simulink model "Quad_Plant_dynamics"  (R2023b)
settings: Solver=FixedStepAuto  StartTime=0.0  StopTime=10.0  RelTol=1e-3
undefined symbols (not defined in the file): altToPrsBias, altToPrsGain, b, battCapacity, c, contact, dragCoeffMov, fractalcoef, g, mass, ms2_to_mg, ms_to_cms, Payload, rotorDir, rotorPositions, rotorThrustMax, rotorTimeConst, rotorTorqueMax, SampleTime, windVel
libraries: simulink x3, uavmavlinklib x3, sharedtransform x2, robotcorelib x2, sensorinslib x1, shared6dof x1, mspsensorlib x1, uavutilslib x1
(part 1 of 2)
settings Model: Creator=The MathWorks, Inc.  LastModifiedBy=LonelyRetard420
settings SolverCC: AlgebraicLoopSolver=TrustRegion
settings OptimizationCC: ReuseModelBlockBuffer=off
settings DebuggingCC: ParameterPrecisionLossMsg=none  UnconnectedInputMsg=warning  UnconnectedOutputMsg=warning  UnconnectedLineMsg=warning
settings ModelReferenceCC: EnableRefExpFcnMdlSchedulingChecks=on  ModelReferenceNumInstancesAllowed=Single
settings RTWCC: DLArmComputeVersion=19.05

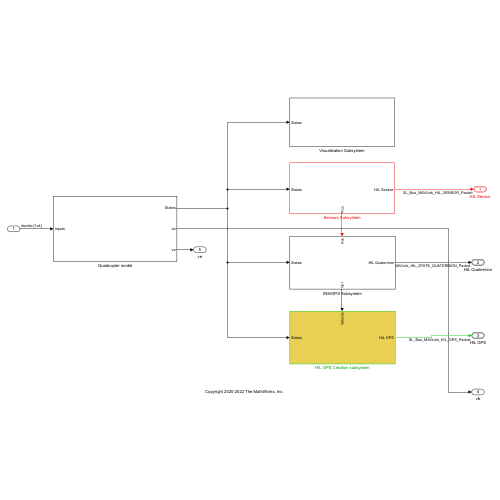
[thumbnail: Simulink's stored preview of the top-level diagram]
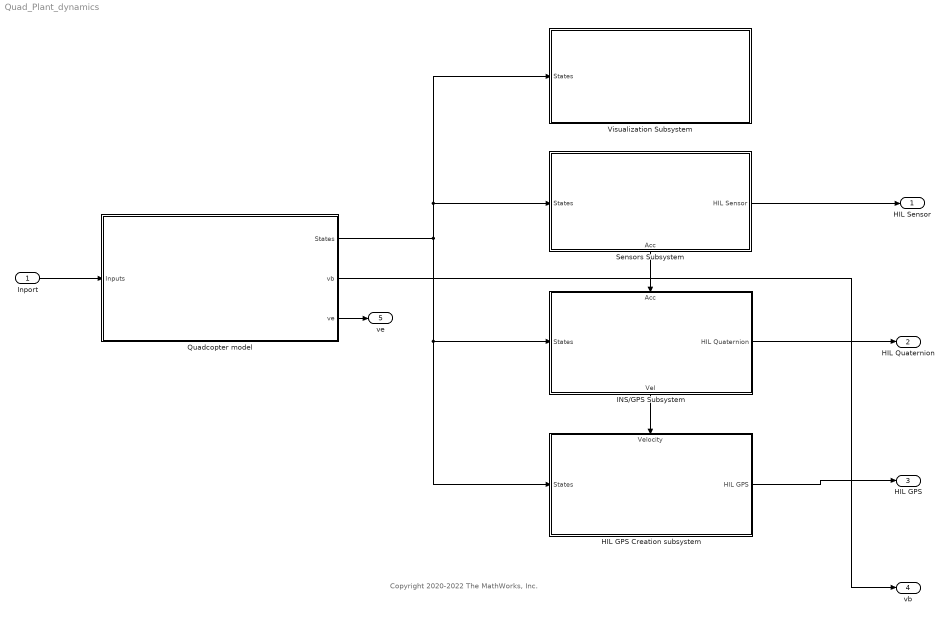
== system Quad_Plant_dynamics ==
  note: Copyright 2020-2022 The MathWorks, Inc.
  Inport : Inport  OutDataTypeStr=double  PortDimensions=[1 4]
  HIL GPS Creation subsystem : Subsystem
      settings: PortSchema="{\"entries\":[{\"content\":{\"sides\":[{\"content\":{\"connectorIds\":[\"In1\"]},\"type\":\"ConnectorPlacement.EquallySpacedRectSide\",\"uuid\":\"f4444677-f205-4bd8-9e95-5e6060697dc4\"},{\"content\":{\"connectorIds\":[\"Out1\"],\"side\":\"RIGHT\"},\"type\":\"ConnectorPlacement.EquallySpacedRectSide\",\"uuid\":\"c948a3e0-826b-4d7b-9e4f-6e3881854d5a\"},{\"content\":{\"connectorIds\":[\"In2\"],\"side\":\"TOP\"},\"type\":\"ConnectorPlacement.EquallySpacedRectSide\",\"uuid\":\"82cf0daf-0b59-4b3c-ab0e-258a514f37ad\"},{\"content\":{\"connectorIds\":[],\"side\":\"HIDDEN\"},\"type\":\"ConnectorPlacement.EquallySpacedRectSide\",\"uuid\":\"a794f320-9150-4c05-acf0-96079b0d3066\"}]},\"type\":\"ConnectorPlacement.EquallySpacedConnector\",\"uuid\":\"8d0915ff-9064-46da-be4f-31886e994f25\"}],\"packageUris\":[\"http://schema.mathworks.com/mf0/Connector/R2020b\"],\"version\":\"1.0\"}"
  INS/GPS Subsystem : Subsystem
      settings: PortSchema="{\"entries\":[{\"content\":{\"sides\":[{\"content\":{\"connectorIds\":[\"In1\"]},\"type\":\"ConnectorPlacement.EquallySpacedRectSide\",\"uuid\":\"bd7d303d-974a-4dd9-8d27-04cf87176bd7\"},{\"content\":{\"connectorIds\":[\"Out1\"],\"side\":\"RIGHT\"},\"type\":\"ConnectorPlacement.EquallySpacedRectSide\",\"uuid\":\"9b60b4cf-af27-4ca7-86b7-e75d27668f15\"},{\"content\":{\"connectorIds\":[\"In2\"],\"side\":\"TOP\"},\"type\":\"ConnectorPlacement.EquallySpacedRectSide\",\"uuid\":\"cd4d20a6-3033-4c65-942d-f02a7fa933e8\"},{\"content\":{\"connectorIds\":[\"Out2\"],\"side\":\"BOTTOM\"},\"type\":\"ConnectorPlacement.EquallySpacedRectSide\",\"uuid\":\"d837ff15-3ee7-4ba9-aab0-0378a7633b3a\"},{\"content\":{\"connectorIds\":[],\"side\":\"HIDDEN\"},\"type\":\"ConnectorPlacement.EquallySpacedRectSide\",\"uuid\":\"eefe2c49-f98f-4c11-8e75-b071b558b610\"}]},\"type\":\"ConnectorPlacement.EquallySpacedConnector\",\"uuid\":\"bd9fca06-cb18-49af-bec9-4d4823ab7b04\"}],\"packageUris\":[\"http://schema.mathworks.com/mf0/Connector/R2020b\"],\"version\":\"1.0\"}"
  Quadcopter model : Subsystem
  Sensors Subsystem : Subsystem
      settings: PortSchema="{\"entries\":[{\"content\":{\"sides\":[{\"content\":{\"connectorIds\":[\"In1\"]},\"type\":\"ConnectorPlacement.EquallySpacedRectSide\",\"uuid\":\"0f5c2282-ad4e-4c27-a92f-532c88dd9b34\"},{\"content\":{\"connectorIds\":[\"Out1\"],\"side\":\"RIGHT\"},\"type\":\"ConnectorPlacement.EquallySpacedRectSide\",\"uuid\":\"b1a389a9-bd19-4f0a-ab56-19663216dbdf\"},{\"content\":{\"connectorIds\":[],\"side\":\"TOP\"},\"type\":\"ConnectorPlacement.EquallySpacedRectSide\",\"uuid\":\"61bb26dd-3b4e-45d7-8996-b1e12f9a0a9d\"},{\"content\":{\"connectorIds\":[\"Out2\"],\"side\":\"BOTTOM\"},\"type\":\"ConnectorPlacement.EquallySpacedRectSide\",\"uuid\":\"ba157af1-2ca4-4452-bdd7-6e3dad9cb5e7\"},{\"content\":{\"connectorIds\":[],\"side\":\"HIDDEN\"},\"type\":\"ConnectorPlacement.EquallySpacedRectSide\",\"uuid\":\"fff182b3-fe96-4082-825e-95746cd3e6b2\"}]},\"type\":\"ConnectorPlacement.EquallySpacedConnector\",\"uuid\":\"8a88afc7-c2a2-4beb-8758-d3390628bed4\"}],\"packageUris\":[\"http://schema.mathworks.com/mf0/Connector/R2020b\"],\"version\":\"1.0\"}"
  Visualization Subsystem : Subsystem
  HIL Sensor : Outport  OutDataTypeStr=Bus: SL_Bus_MAVLink_HIL_SENSOR_Packet  BusOutputAsStruct=on
  HIL Quaternion : Outport  Port=2  OutDataTypeStr=Bus: SL_Bus_MAVLink_HIL_STATE_QUATERNION_Packet  BusOutputAsStruct=on
  HIL GPS : Outport  Port=3  OutDataTypeStr=Bus: SL_Bus_MAVLink_HIL_GPS_Packet  BusOutputAsStruct=on
  vb : Outport  Port=4
  ve : Outport  Port=5
  wires:
  Sensors Subsystem/1(HIL Sensor) -> HIL Sensor/1
  HIL GPS Creation subsystem/1(HIL GPS) -> HIL GPS/1
  INS/GPS Subsystem/2(Vel) -> HIL GPS Creation subsystem/2(Velocity)
  Quadcopter model/1(States) -> HIL GPS Creation subsystem/1(States), INS/GPS Subsystem/1(States), Visualization Subsystem/1(States), Sensors Subsystem/1(States)
  Sensors Subsystem/2(Acc) -> INS/GPS Subsystem/2(Acc)
  Inport/1 -> Quadcopter model/1(Inputs)
  INS/GPS Subsystem/1(HIL Quaternion) -> HIL Quaternion/1
  Quadcopter model/2(vb) -> vb/1
  Quadcopter model/3(ve) -> ve/1

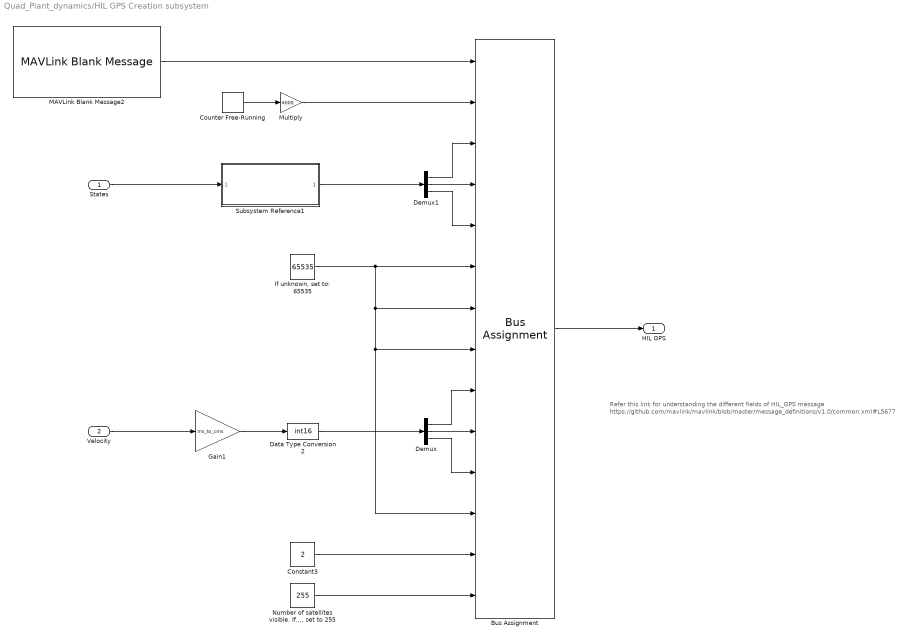
== system Quad_Plant_dynamics/HIL GPS Creation subsystem ==
  note: Refer this link for understanding the different fields of HIL_GPS message https://github.com/mavlink/mavlink/blob/master/message_definitions/v1.0/common.xml#L5677
  States : Inport
  Velocity : Inport  Port=2
  Bus Assignment : BusAssignment  AssignedSignals=Payload.time_usec,Payload.lat,Payload.lon,Payload.alt,Payload.eph,Payload.epv,Payload.vel,Payload.vn,Payload.ve,Payload.vd,Payload.cog,Payload.fix_type,Payload.satellites_visible
  Constant3 : Constant  Value=2  OutDataTypeStr=Inherit: Inherit via back propagation
  Counter Free-Running : simulink/Sources/Counter Free-Running  NumBits=64  tsamp=-1
  Data Type Conversion2 : DataTypeConversion  OutDataTypeStr=int16  SaturateOnIntegerOverflow=off  RndMeth=Floor
  Demux : Demux  Outputs=3
  Demux1 : Demux  Outputs=3
  Gain1 : Gain  Gain=ms_to_cms
  "If unknown, set to: 65535" : Constant  Value=65535  OutDataTypeStr=Inherit: Inherit via back propagation
  MAVLink Blank Message2 : uavmavlinklib/MAVLink Blank Message  dialectSource=Select from standard MAVLink dialects  dialect=common.xml  dialectCustom=common.xml  version=2  messageType=HIL_GPS  SystemID=2  ComponentID=51  SampleTime=SampleTime
  Multiply : Gain  Gain=4000  OutDataTypeStr=Inherit: Inherit via back propagation
  "Number of satellites visible. If unknown, set to 255" : Constant  Value=255  OutDataTypeStr=Inherit: Inherit via back propagation
  Subsystem Reference1 : Subsystem  ReferencedSubsystem=Create_LLA_from_States
  HIL GPS : Outport
  wires:
  MAVLink Blank Message2/1 -> Bus Assignment/1
  Counter Free-Running/1 -> Multiply/1
  Multiply/1 -> Bus Assignment/2
  Bus Assignment/1 -> HIL GPS/1
  "Number of satellites visible. If unknown, set to 255"/1 -> Bus Assignment/14
  "If unknown, set to: 65535"/1 -> Bus Assignment/12, Bus Assignment/8, Bus Assignment/7, Bus Assignment/6
  Constant3/1 -> Bus Assignment/13
  Gain1/1 -> Data Type Conversion2/1
  Velocity/1 -> Gain1/1
  Data Type Conversion2/1 -> Demux/1
  Demux/2 -> Bus Assignment/10
  Demux/1 -> Bus Assignment/9
  Demux/3 -> Bus Assignment/11
  States/1 -> Subsystem Reference1/1
  Demux1/3 -> Bus Assignment/5
  Demux1/2 -> Bus Assignment/4
  Demux1/1 -> Bus Assignment/3
  Subsystem Reference1/1 -> Demux1/1

== system Quad_Plant_dynamics/INS//GPS Subsystem ==
  States : Inport
  Acc : Inport  Port=2
  HIL Quaternion Creation Subsystem : Subsystem
  INS : Subsystem
  HIL Quaternion : Outport
  Vel : Outport  Port=2
  wires:
  HIL Quaternion Creation Subsystem/1(HIL Quaternion) -> HIL Quaternion/1
  States/1 -> HIL Quaternion Creation Subsystem/2(States), INS/1(States)
  Acc/1 -> HIL Quaternion Creation Subsystem/1(Acc)
  INS/1(Vel) -> Vel/1

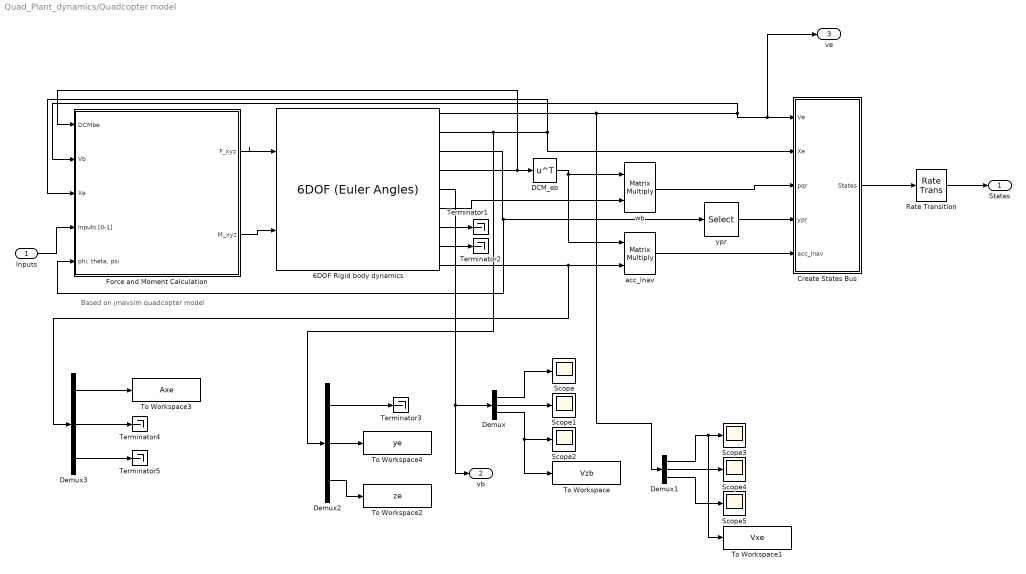
== system Quad_Plant_dynamics/Quadcopter model ==
  note: Based on jmavsim quadcopter model
  Inputs : Inport
  "6DOF Rigid body dynamics " : shared6dof/6DOF (Euler Angles)  units=Metric (MKS)  mtype=Fixed  rep=Euler Angles  xme_0=init.posNED  Vm_0=init.vb  eul_0=init.euler  pm_0=init.angRates  mass_0=mass  mass_e=0.5  mass_f=2.0  inertia=inertia  inertia_e=eye(3)  inertia_f=2*eye(3)  k_quat=Vehicle.SixDOF.quatGain  vre_flag=on  abi_flag=on  aMode=aMode  xme_statename=''  Vm_statename=''  eul_statename=''  quat_statename=''  pm_statename=''  mass_statename=''
  Create States Bus : Subsystem
  DCM_eb : Math  Operator=transpose
  Demux{,1..3} (4 alike) : Demux  Outputs=3
  Force and Moment Calculation : Subsystem
  Rate Transition : RateTransition  OutPortSampleTime=SampleTime
  Scope{,1..5} (6 alike) : Scope
  Terminator{1..5} (5 alike) : Terminator
  To Workspace : ToWorkspace  VariableName=Vzb  SampleTime=-1
  To Workspace1 : ToWorkspace  VariableName=Vxe  SampleTime=-1
  To Workspace2 : ToWorkspace  VariableName=ze  SaveFormat=Timeseries  SampleTime=-1
  To Workspace3 : ToWorkspace  VariableName=Axe  SaveFormat=Timeseries  SampleTime=-1
  To Workspace4 : ToWorkspace  VariableName=ye  SampleTime=-1
  acc_lnav : Product  Multiplication=Matrix(*)
  wb : Product  Multiplication=Matrix(*)
  ypr : Selector  InputPortWidth=3  IndexOptions=Index vector (dialog)  Indices=[3 2 1]  OutputSizes=1
  States : Outport
  vb : Outport  Port=2
  ve : Outport  Port=3
  wires:
  "6DOF Rigid body dynamics "/3 -> Force and Moment Calculation/5("phi, theta, psi"), ypr/1
  Force and Moment Calculation/1(F_xyz) -> "6DOF Rigid body dynamics "/1
  Force and Moment Calculation/2(M_xyz) -> "6DOF Rigid body dynamics "/2
  Rate Transition/1 -> States/1
  "6DOF Rigid body dynamics "/1 -> Force and Moment Calculation/2(Vb), ve/1, Create States Bus/1(Ve), Demux1/1
  Inputs/1 -> Force and Moment Calculation/4(Inputs [0-1])
  ypr/1 -> Create States Bus/4(ypr)
  Create States Bus/1(States) -> Rate Transition/1
  "6DOF Rigid body dynamics "/4 -> DCM_eb/1, Force and Moment Calculation/1(DCMbe)
  "6DOF Rigid body dynamics "/2 -> Demux2/1, Force and Moment Calculation/3(Xe), Create States Bus/2(Xe)
  "6DOF Rigid body dynamics "/6 -> wb/2
  wb/1 -> Create States Bus/3(pqr)
  DCM_eb/1 -> acc_lnav/1, wb/1
  "6DOF Rigid body dynamics "/9 -> Demux3/1, acc_lnav/2
  acc_lnav/1 -> Create States Bus/5(acc_lnav)
  "6DOF Rigid body dynamics "/5 -> vb/1, Demux/1
  "6DOF Rigid body dynamics "/7 -> Terminator1/1
  "6DOF Rigid body dynamics "/8 -> Terminator2/1
  Demux/2 -> Scope1/1
  Demux/1 -> Scope/1
  Demux/3 -> To Workspace/1, Scope2/1
  Demux1/2 -> Scope4/1
  Demux1/3 -> Scope5/1
  Demux1/1 -> To Workspace1/1, Scope3/1
  Demux2/3 -> To Workspace2/1
  Demux2/1 -> Terminator3/1
  Demux3/1 -> To Workspace3/1
  Demux3/2 -> Terminator4/1
  Demux3/3 -> Terminator5/1
  Demux2/2 -> To Workspace4/1

== system Quad_Plant_dynamics/Sensors Subsystem ==
  States : Inport
  Hil Sensor Creation subsystem : Subsystem
  IMU Subsystem : Subsystem
  HIL Sensor : Outport
  Acc : Outport  Port=2
  wires:
  States/1 -> Hil Sensor Creation subsystem/4(States), IMU Subsystem/1(States)
  Hil Sensor Creation subsystem/1(HIL Sensor) -> HIL Sensor/1
  IMU Subsystem/2(Gyro) -> Hil Sensor Creation subsystem/2(Gyro)
  IMU Subsystem/1(Acc) -> Acc/1, Hil Sensor Creation subsystem/1(Acc)
  IMU Subsystem/3(Mag) -> Hil Sensor Creation subsystem/3(Mag)

== system Quad_Plant_dynamics/Visualization Subsystem ==
  States : Inport
  Bus Selector : BusSelector  OutputSignals=X,Y,Z  OutputAsBus=on
  Bus Selector1 : BusSelector  OutputSignals=yaw,pitch,roll  OutputAsBus=on
  Rotation Angles to Quaternions : sharedtransform/Rotation Angles to Quaternions  rotationOrder=ZYX  aMode=aMode
  UAV Animation : uavutilslib/UAV Animation  UAVType=Multirotor  UAVSize=1  InertialZDirection=Down  SampleTime=-1
  wires:
  Bus Selector/1 -> UAV Animation/1
  Rotation Angles to Quaternions/1 -> UAV Animation/2
  Bus Selector1/1 -> Rotation Angles to Quaternions/1
  States/1 -> Bus Selector1/1, Bus Selector/1

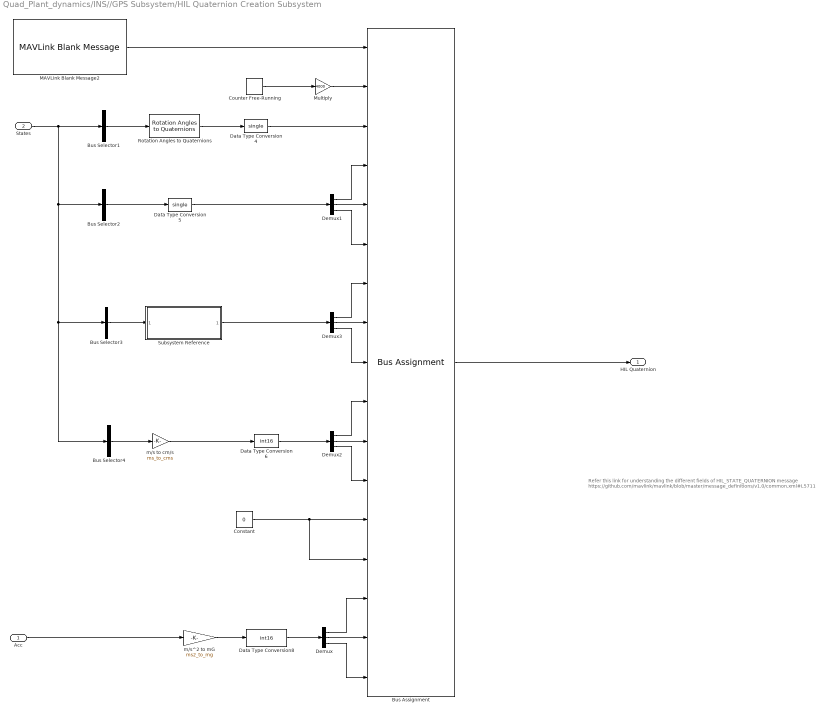
== system Quad_Plant_dynamics/INS//GPS Subsystem/HIL Quaternion Creation Subsystem ==
  note: Refer this link for understanding the different fields of HIL_STATE_QUATERNION message https://github.com/mavlink/mavlink/blob/master/message_definitions/v1.0/common.xml#L5711
  Acc : Inport
  States : Inport  Port=2
  Bus Assignment : BusAssignment  AssignedSignals=Payload.time_usec,Payload.attitude_quaternion,Payload.rollspeed,Payload.pitchspeed,Payload.yawspeed,Payload.lat,Payload.lon,Payload.alt,Payload.vx,Payload.vy,Payload.vz,Payload.ind_airspeed,Payload.true_airspeed,Payload.xacc,Payload.yacc,Payload.zacc
  Bus Selector1 : BusSelector  OutputSignals=yaw,pitch,roll  OutputAsBus=on
  Bus Selector2 : BusSelector  OutputSignals=r,q,p  OutputAsBus=on
  Bus Selector3 : BusSelector  OutputSignals=X,Y,Z  OutputAsBus=on
  Bus Selector4 : BusSelector  OutputSignals=dx,dy,dz  OutputAsBus=on
  Constant : Constant  Value=0  OutDataTypeStr=Inherit: Inherit via back propagation
  Counter Free-Running : simulink/Sources/Counter Free-Running  NumBits=64  tsamp=-1
  Data Type Conversion4 : DataTypeConversion  OutDataTypeStr=single  SaturateOnIntegerOverflow=off  RndMeth=Floor
  Data Type Conversion5 : DataTypeConversion  OutDataTypeStr=single  SaturateOnIntegerOverflow=off  RndMeth=Floor
  Data Type Conversion6 : DataTypeConversion  OutDataTypeStr=int16  SaturateOnIntegerOverflow=off  RndMeth=Floor
  Data Type Conversion8 : DataTypeConversion  OutDataTypeStr=int16  SaturateOnIntegerOverflow=off  RndMeth=Floor
  Demux{,1..3} (4 alike) : Demux  Outputs=3
  MAVLink Blank Message2 : uavmavlinklib/MAVLink Blank Message  dialectSource=Select from standard MAVLink dialects  dialect=common.xml  dialectCustom=common.xml  version=2  messageType=HIL_STATE_QUATERNION  SystemID=2  ComponentID=51  SampleTime=SampleTime
  Multiply : Gain  Gain=4000  OutDataTypeStr=Inherit: Inherit via back propagation
  Rotation Angles to Quaternions : sharedtransform/Rotation Angles to Quaternions  rotationOrder=ZYX  aMode=aMode
  Subsystem Reference : Subsystem  ReferencedSubsystem=Create_LLA_from_States
  m/s to cm/s : Gain  Gain=ms_to_cms
  m/s^2 to mG : Gain  Gain=ms2_to_mg
  HIL Quaternion : Outport
  wires:
  Counter Free-Running/1 -> Multiply/1
  MAVLink Blank Message2/1 -> Bus Assignment/1
  Multiply/1 -> Bus Assignment/2
  Bus Assignment/1 -> HIL Quaternion/1
  States/1 -> Bus Selector1/1, Bus Selector2/1, Bus Selector4/1, Bus Selector3/1
  Rotation Angles to Quaternions/1 -> Data Type Conversion4/1
  Data Type Conversion4/1 -> Bus Assignment/3
  Demux/3 -> Bus Assignment/17
  Demux/1 -> Bus Assignment/15
  Demux/2 -> Bus Assignment/16
  Constant/1 -> Bus Assignment/14, Bus Assignment/13
  m/s to cm/s/1 -> Data Type Conversion6/1
  Data Type Conversion6/1 -> Demux2/1
  Demux2/3 -> Bus Assignment/12
  Demux2/2 -> Bus Assignment/11
  Demux2/1 -> Bus Assignment/10
  Subsystem Reference/1 -> Demux3/1
  Demux3/1 -> Bus Assignment/7
  Demux3/2 -> Bus Assignment/8
  Demux3/3 -> Bus Assignment/9
  Data Type Conversion8/1 -> Demux/1
  Acc/1 -> m/s^2 to mG/1
  m/s^2 to mG/1 -> Data Type Conversion8/1
  Bus Selector1/1 -> Rotation Angles to Quaternions/1
  Data Type Conversion5/1 -> Demux1/1
  Demux1/3 -> Bus Assignment/6
  Demux1/2 -> Bus Assignment/5
  Demux1/1 -> Bus Assignment/4
  Bus Selector2/1 -> Data Type Conversion5/1
  Bus Selector3/1 -> Subsystem Reference/1
  Bus Selector4/1 -> m/s to cm/s/1

== system Quad_Plant_dynamics/INS//GPS Subsystem/INS ==
  States : Inport
  Bus Selector : BusSelector  OutputSignals=X,Y,Z  OutputAsBus=on
  Bus Selector1 : BusSelector  OutputSignals=dx,dy,dz  OutputAsBus=on
  Bus Selector2 : BusSelector  OutputSignals=yaw,pitch,roll  OutputAsBus=on
  Coordinate Transformation Conversion : robotcorelib/Coordinate Transformation Conversion  InputRepresentation=Euler Angles  InputEulerSequence=ZYX  ShowTrVecInputPort=on  OutputRepresentation=Quaternion  OutputEulerSequence=ZYX  ShowTrVecOutputPort=on  SimulateUsing=Interpreted execution
  INS : sensorinslib/INS  MountingLocation=[0 0 0]  RollAccuracy=0.2  PitchAccuracy=0.2  YawAccuracy=1  PositionAccuracy=1  VelocityAccuracy=0.05  UseAccelAndAngVel=off  AccelerationAccuracy=0  AngularVelocityAccuracy=0  TimeInput=off  PositionErrorFactor=[0 0 0]  SeedDouble=67  SimulateUsing=Interpreted execution
  Reshape1 : Reshape  OutputDimensionality=Row vector (2-D)
  Reshape2 : Reshape  OutputDimensionality=Row vector (2-D)
  Reshape3 : Reshape  OutputDimensionality=Row vector (2-D)
  Terminator : Terminator
  Terminator1 : Terminator
  Vel : Outport
  wires:
  Bus Selector1/1 -> Reshape3/1
  Bus Selector/1 -> Reshape2/1
  Reshape2/1 -> INS/1
  Bus Selector2/1 -> Coordinate Transformation Conversion/1
  Reshape3/1 -> INS/2
  States/1 -> Bus Selector2/1, Bus Selector1/1, Bus Selector/1
  Coordinate Transformation Conversion/1 -> Reshape1/1
  INS/1 -> Terminator1/1
  INS/3 -> Terminator/1
  INS/2 -> Vel/1
  Reshape1/1 -> INS/3

== system Quad_Plant_dynamics/Quadcopter model/Create States Bus ==
  Ve : Inport
  Xe : Inport  Port=2
  pqr : Inport  Port=3
  ypr : Inport  Port=4
  acc_lnav : Inport  Port=5
  Bus Creator : BusCreator  Inputs=15
  Demux{,1..4} (5 alike) : Demux  Outputs=3
  States : Outport
  wires:
  Demux1/1 -> Bus Creator/1  "X"
  Demux1/2 -> Bus Creator/2  "Y"
  ypr/1 -> Demux2/1
  Demux2/2 -> Bus Creator/5  "pitch"
  Demux3/2 -> Bus Creator/8  "dy"
  Demux2/3 -> Bus Creator/6  "roll"
  pqr/1 -> Demux4/1
  Ve/1 -> Demux3/1
  Demux2/1 -> Bus Creator/4  "yaw"
  Demux1/3 -> Bus Creator/3  "Z"
  Demux3/1 -> Bus Creator/7  "dx"
  Demux4/2 -> Bus Creator/11  "q"
  Demux3/3 -> Bus Creator/9  "dz"
  Demux4/3 -> Bus Creator/12  "r"
  Demux4/1 -> Bus Creator/10  "p"
  Bus Creator/1 -> States/1
  Xe/1 -> Demux1/1
  acc_lnav/1 -> Demux/1
  Demux/3 -> Bus Creator/15  "ddz"
  Demux/2 -> Bus Creator/14  "ddy"
  Demux/1 -> Bus Creator/13  "ddx"

== system Quad_Plant_dynamics/Quadcopter model/Force and Moment Calculation ==
  DCMbe : Inport
  Vb : Inport  Port=2
  Xe : Inport  Port=3
  Inputs [0-1] : Inport  Port=4
  "phi, theta, psi" : Inport  Port=5
  Add : Sum  Inputs=++++
  Aerodynamic drag : Subsystem
  Demux1 : Demux  Outputs=3
  Gravity : Subsystem
  Ground Model : Subsystem
  Rotor Model : Subsystem
  To Workspace4 : ToWorkspace  VariableName=Fz  SaveFormat=Timeseries  SampleTime=-1
  F_xyz : Outport
  M_xyz : Outport  Port=2
  wires:
  Inputs [0-1]/1 -> Rotor Model/1(Inputs [0-1])
  Gravity/1(F_g) -> Add/1
  Rotor Model/2(M_rotors) -> M_xyz/1
  Rotor Model/1(F_rotors) -> Add/2
  Aerodynamic drag/1(F_d) -> Add/3
  Ground Model/1(Fb_contact) -> Add/4
  Vb/1 -> Rotor Model/2(vb), Aerodynamic drag/2(Vb), Ground Model/3(Vb)
  DCMbe/1 -> Ground Model/1(DCMbe), Aerodynamic drag/1(DCMbe), Gravity/1(DCM_be)
  Xe/1 -> Ground Model/2(Xe)
  "phi, theta, psi"/1 -> Rotor Model/3("phi, theta, psi")
  Add/1 -> Demux1/1, F_xyz/1
  Demux1/3 -> To Workspace4/1

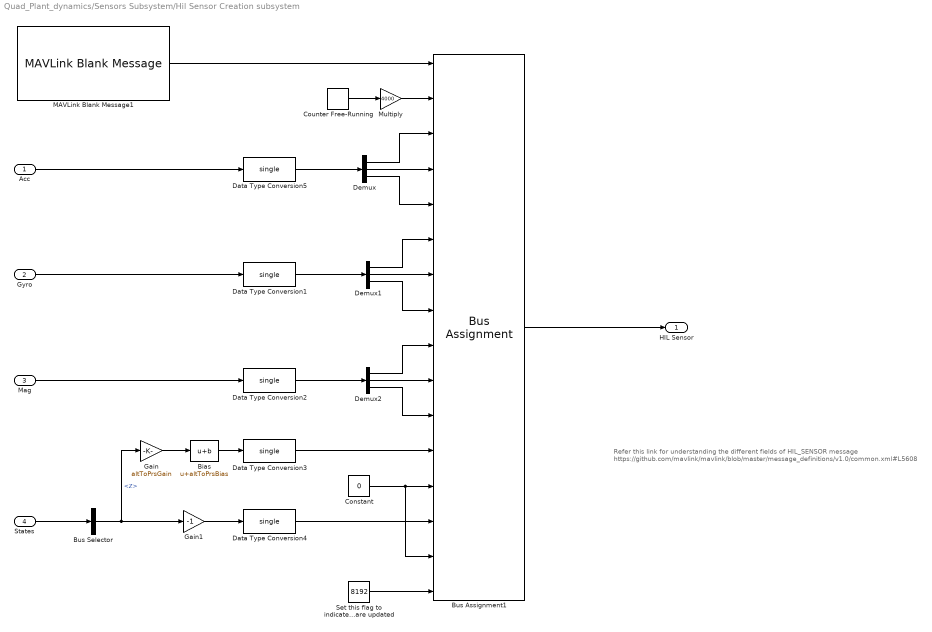
== system Quad_Plant_dynamics/Sensors Subsystem/Hil Sensor Creation subsystem ==
  note: Refer this link for understanding the different fields of HIL_SENSOR message https://github.com/mavlink/mavlink/blob/master/message_definitions/v1.0/common.xml#L5608
  Acc : Inport
  Gyro : Inport  Port=2
  Mag : Inport  Port=3
  States : Inport  Port=4
  Bias : Bias  Bias=altToPrsBias  SaturateOnIntegerOverflow=off
  Bus Assignment1 : BusAssignment  AssignedSignals=Payload.time_usec,Payload.xacc,Payload.yacc,Payload.zacc,Payload.xgyro,Payload.ygyro,Payload.zgyro,Payload.xmag,Payload.ymag,Payload.zmag,Payload.abs_pressure,Payload.diff_pressure,Payload.pressure_alt,Payload.temperature,Payload.fields_updated
  Bus Selector : BusSelector  OutputSignals=Z
  Constant : Constant  Value=0  OutDataTypeStr=Inherit: Inherit via back propagation  SampleTime=SampleTime
  Counter Free-Running : simulink/Sources/Counter Free-Running  NumBits=64  tsamp=SampleTime
  Data Type Conversion{1..5} (5 alike) : DataTypeConversion  OutDataTypeStr=single  SaturateOnIntegerOverflow=off  RndMeth=Floor
  Demux : Demux  Outputs=3
  Demux1 : Demux  Outputs=3
  Demux2 : Demux  Outputs=3
  Gain : Gain  Gain=altToPrsGain
  Gain1 : Gain  Gain=-1
  MAVLink Blank Message1 : uavmavlinklib/MAVLink Blank Message  dialectSource=Select from standard MAVLink dialects  dialect=common.xml  dialectCustom=common.xml  version=2  messageType=HIL_SENSOR  SystemID=2  ComponentID=51  SampleTime=SampleTime
  Multiply : Gain  Gain=4000  OutDataTypeStr=Inherit: Inherit via back propagation
  Set this flag to indicate all flags are updated : Constant  Value=8192  OutDataTypeStr=Inherit: Inherit via back propagation  SampleTime=SampleTime
  HIL Sensor : Outport
  wires:
  Data Type Conversion2/1 -> Demux2/1
  Demux1/1 -> Bus Assignment1/6
  Counter Free-Running/1 -> Multiply/1
  Mag/1 -> Data Type Conversion2/1
  Demux1/3 -> Bus Assignment1/8
  Data Type Conversion1/1 -> Demux1/1
  Gyro/1 -> Data Type Conversion1/1
  Bus Assignment1/1 -> HIL Sensor/1
  Set this flag to indicate all flags are updated/1 -> Bus Assignment1/16
  Demux/3 -> Bus Assignment1/5
  Demux2/2 -> Bus Assignment1/10
  Demux2/3 -> Bus Assignment1/11
  Data Type Conversion5/1 -> Demux/1
  Demux/1 -> Bus Assignment1/3
  Multiply/1 -> Bus Assignment1/2
  Constant/1 -> Bus Assignment1/15, Bus Assignment1/13
  MAVLink Blank Message1/1 -> Bus Assignment1/1
  Demux2/1 -> Bus Assignment1/9
  Demux/2 -> Bus Assignment1/4
  Demux1/2 -> Bus Assignment1/7
  Bus Selector/1 -> Gain/1, Gain1/1  "<Z>"
  Acc/1 -> Data Type Conversion5/1
  States/1 -> Bus Selector/1
  Bias/1 -> Data Type Conversion3/1
  Gain/1 -> Bias/1
  Data Type Conversion4/1 -> Bus Assignment1/14
  Data Type Conversion3/1 -> Bus Assignment1/12
  Gain1/1 -> Data Type Conversion4/1

== system Quad_Plant_dynamics/Sensors Subsystem/IMU Subsystem ==
  States : Inport
  Bus Selector1 : BusSelector  OutputSignals=p,q,r  OutputAsBus=on
  Bus Selector2 : BusSelector  OutputSignals=yaw,pitch,roll  OutputAsBus=on
  Bus Selector3 : BusSelector  OutputSignals=ddx,ddy,ddz  OutputAsBus=on
  Coordinate Transformation Conversion1 : robotcorelib/Coordinate Transformation Conversion  InputRepresentation=Euler Angles  InputEulerSequence=ZYX  ShowTrVecInputPort=on  OutputRepresentation=Quaternion  OutputEulerSequence=ZYX  ShowTrVecOutputPort=on  SimulateUsing=Interpreted execution
  Gain : Gain  Gain=-1
  IMU : mspsensorlib/IMU  DispRefFrame=NED  TemperaturePort=off  Temperature=25  MagneticFieldPort=off  MagneticFieldNED=[ 27.5550, -2.4169, -16.0849 ]  MagneticFieldENU=[ -2.4169, 27.5550, 16.0849 ]  SeedDouble=67  SimulateUsing=Interpreted execution  AccelParamsMeasurementRange=Inf  AccelParamsResolution=0  AccelParamsConstantBias=[ 0, 0, 0 ]  AccelParamsAxesMisalignment=[ 0, 0, 0 ]  AccelParamsNoiseDensity=[ 0, 0, 0 ]  AccelParamsBiasInstability=[ 0, 0, 0 ]  AccelParamsBiasInstabilityNumerator=fractalcoef().Numerator  AccelParamsBiasInstabilityDenominator=fractalcoef().Denominator  AccelParamsRandomWalk=[ 0, 0, 0 ]  AccelParamsNoiseType=double-sided  AccelParamsTemperatureBias=[ 0, 0, 0 ]  AccelParamsTemperatureScaleFactor=[ 0, 0, 0 ]  GyroParamsMeasurementRange=Inf  GyroParamsResolution=0  GyroParamsConstantBias=[ 0, 0, 0 ]  GyroParamsAxesMisalignment=[ 0, 0, 0 ]  GyroParamsAccelerationBias=[ 0, 0, 0 ]  GyroParamsNoiseDensity=[ 0, 0, 0 ]  GyroParamsBiasInstability=[ 0, 0, 0 ]  GyroParamsBiasInstabilityNumerator=fractalcoef().Numerator  GyroParamsBiasInstabilityDenominator=fractalcoef().Denominator  GyroParamsRandomWalk=[ 0, 0, 0 ]  GyroParamsNoiseType=double-sided  GyroParamsTemperatureBias=[ 0, 0, 0 ]  GyroParamsTemperatureScaleFactor=[ 0, 0, 0 ]  MagParamsMeasurementRange=Inf  MagParamsResolution=0  MagParamsConstantBias=[ 0, 0, 0 ]  MagParamsAxesMisalignment=[ 0, 0, 0 ]  MagParamsNoiseDensity=[ 0, 0, 0 ]  MagParamsBiasInstability=[ 0, 0, 0 ]  MagParamsBiasInstabilityNumerator=fractalcoef().Numerator  MagParamsBiasInstabilityDenominator=fractalcoef().Denominator  MagParamsRandomWalk=[ 0, 0, 0 ]  MagParamsNoiseType=double-sided  MagParamsTemperatureBias=[ 0, 0, 0 ]  MagParamsTemperatureScaleFactor=[ 0, 0, 0 ]
  Reshape : Reshape  OutputDimensionality=Row vector (2-D)
  Reshape2 : Reshape  OutputDimensionality=Row vector (2-D)
  Reshape3 : Reshape  OutputDimensionality=Row vector (2-D)
  Acc : Outport
  Gyro : Outport  Port=2
  Mag : Outport  Port=3
  wires:
  Bus Selector1/1 -> Reshape2/1
  IMU/1 -> Gain/1
  Bus Selector2/1 -> Coordinate Transformation Conversion1/1
  IMU/3 -> Mag/1
  Reshape2/1 -> IMU/2
  Bus Selector3/1 -> Reshape/1
  Coordinate Transformation Conversion1/1 -> Reshape3/1
  Reshape/1 -> IMU/1
  IMU/2 -> Gyro/1
  Reshape3/1 -> IMU/3
  States/1 -> Bus Selector3/1, Bus Selector2/1, Bus Selector1/1
  Gain/1 -> Acc/1

== system Quad_Plant_dynamics/Quadcopter model/Force and Moment Calculation/Aerodynamic drag ==
  DCMbe : Inport
  Vb : Inport  Port=2
  Constant : Constant  Value=windVel
  Constant1 : Constant  Value=dragCoeffMov
  calcDragVector : MATLAB Function  TreatAsAtomicUnit=on
  gain : Gain  Gain=-1
  relative air velocity (body frame) : Sum
  wind (body frame) : Product  Commented=on  Multiplication=Matrix(*)
  F_d : Outport
  wires:
  Vb/1 -> gain/1
  calcDragVector/1(dragVec) -> F_d/1
  relative air velocity (body frame)/1 -> calcDragVector/1(airVel)
  gain/1 -> relative air velocity (body frame)/2
  Constant1/1 -> calcDragVector/2(dragCoeff)
  DCMbe/1 -> wind (body frame)/1
  Constant/1 -> relative air velocity (body frame)/1

== system Quad_Plant_dynamics/Quadcopter model/Force and Moment Calculation/Gravity ==
  DCM_be : Inport
  Constant : Constant  Value=[0 0 g]'
  Gain : Gain  Gain=mass
  Matrix Multiply : Product  Commented=on  Multiplication=Matrix(*)
  Scope : Scope
  To Workspace : ToWorkspace  VariableName=FG  SampleTime=-1
  F_g : Outport
  wires:
  Gain/1 -> To Workspace/1, Scope/1, F_g/1
  DCM_be/1 -> Matrix Multiply/1
  Constant/1 -> Gain/1

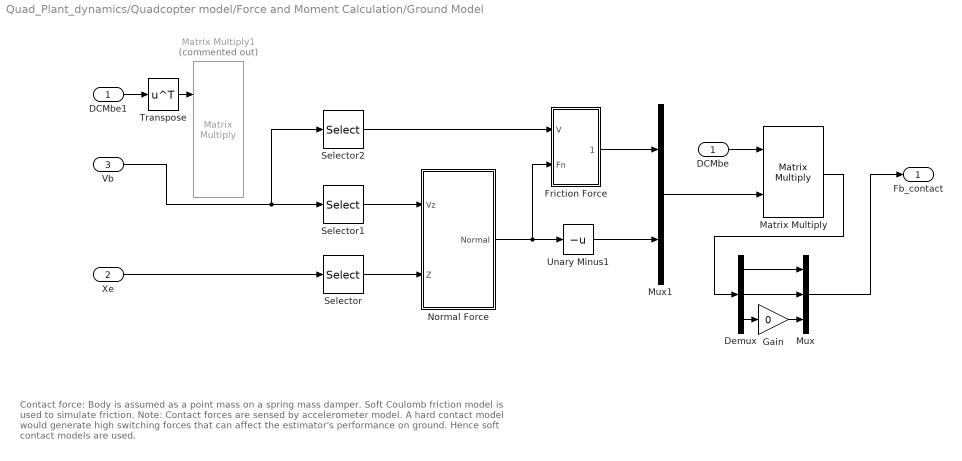
== system Quad_Plant_dynamics/Quadcopter model/Force and Moment Calculation/Ground Model ==
  note: Contact force:
      | Body is assumed as a point mass on a spring mass damper. Soft Coulomb friction model is used to simulate friction.
      |
      | Note:
      | Contact forces are sensed by accelerometer model. A hard contact model would generate high switching forces that can affect the estimator's performance on ground. Hence soft contact models are used.
  DCMbe : Inport
  Xe : Inport  Port=2
  Vb : Inport  Port=3
  DCMbe1 : InportShadow
  Demux : Demux  Outputs=3
  Friction Force : Subsystem
  Gain : Gain  Gain=0
  Matrix Multiply : Product  Multiplication=Matrix(*)
  Matrix Multiply1 : Product  Commented=on  Multiplication=Matrix(*)
  Mux : Mux  Inputs=3
  Mux1 : Mux  Inputs=2
  Normal Force : Subsystem
  Selector : Selector  InputPortWidth=3  IndexOptions=Index vector (dialog)  Indices=[3]  OutputSizes=1
  Selector1 : Selector  InputPortWidth=3  IndexOptions=Index vector (dialog)  Indices=[3]  OutputSizes=1
  Selector2 : Selector  InputPortWidth=3  IndexOptions=Index vector (dialog)  Indices=[1,2]  OutputSizes=1
  Transpose : Math  Operator=transpose
  Unary Minus1 : UnaryMinus
  Fb_contact : Outport
  wires:
  Xe/1 -> Selector/1
  Selector1/1 -> Normal Force/1(Vz)
  Selector/1 -> Normal Force/2(Z)
  DCMbe/1 -> Matrix Multiply/1
  Matrix Multiply/1 -> Demux/1
  Normal Force/1(Normal) -> Unary Minus1/1, Friction Force/2(Fn)
  Unary Minus1/1 -> Mux1/2
  Selector2/1 -> Friction Force/1(V)
  Friction Force/1(Friction) -> Mux1/1
  DCMbe1/1 -> Transpose/1
  Transpose/1 -> Matrix Multiply1/1
  Demux/3 -> Gain/1
  Gain/1 -> Mux/3
  Demux/2 -> Mux/2
  Demux/1 -> Mux/1
  Mux1/1 -> Matrix Multiply/2
  Mux/1 -> Fb_contact/1
  Vb/1 -> Selector2/1, Selector1/1

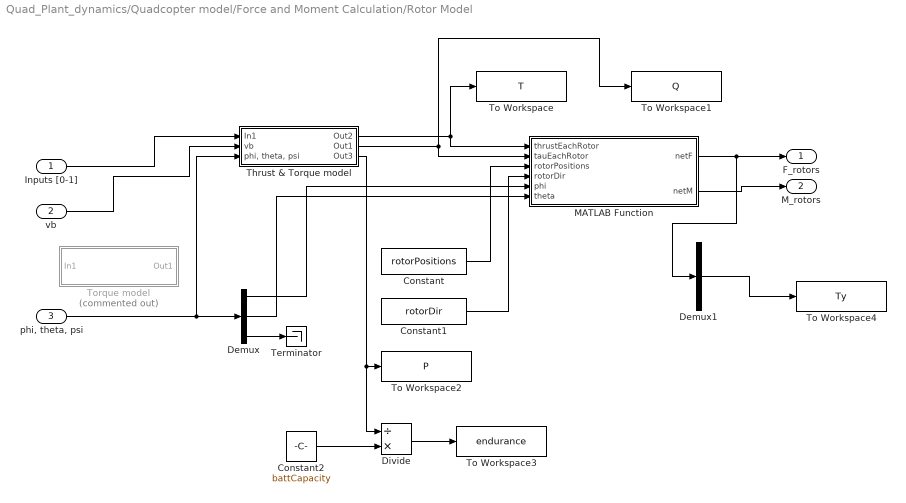
== system Quad_Plant_dynamics/Quadcopter model/Force and Moment Calculation/Rotor Model ==
  Inputs [0-1] : Inport
  vb : Inport  Port=2
  "phi, theta, psi" : Inport  Port=3
  Constant : Constant  Value=rotorPositions
  Constant1 : Constant  Value=rotorDir
  Constant2 : Constant  Value=battCapacity
  Demux : Demux  Outputs=3
  Demux1 : Demux  Outputs=3
  Divide : Product  Inputs=/*
  MATLAB Function : MATLAB Function  TreatAsAtomicUnit=on
  Terminator : Terminator
  Thrust & Torque model : Subsystem
  To Workspace : ToWorkspace  VariableName=T  SampleTime=-1
  To Workspace1 : ToWorkspace  VariableName=Q  SaveFormat=Timeseries  SampleTime=-1
  To Workspace2 : ToWorkspace  VariableName=P  SaveFormat=Timeseries  SampleTime=-1
  To Workspace3 : ToWorkspace  VariableName=endurance  SampleTime=-1
  To Workspace4 : ToWorkspace  VariableName=Ty  SaveFormat=Timeseries  SampleTime=-1
  Torque model : Subsystem  Commented=on
  F_rotors : Outport
  M_rotors : Outport  Port=2
  wires:
  Inputs [0-1]/1 -> Thrust & Torque model/1(In1)
  MATLAB Function/1(netF) -> Demux1/1, F_rotors/1
  MATLAB Function/2(netM) -> M_rotors/1
  Constant/1 -> MATLAB Function/3(rotorPositions)
  Constant1/1 -> MATLAB Function/4(rotorDir)
  Thrust & Torque model/2(Out1) -> MATLAB Function/2(tauEachRotor), To Workspace1/1
  Thrust & Torque model/1(Out2) -> MATLAB Function/1(thrustEachRotor), To Workspace/1
  vb/1 -> Thrust & Torque model/2(vb)
  "phi, theta, psi"/1 -> Demux/1, Thrust & Torque model/3("phi, theta, psi")
  Thrust & Torque model/3(Out3) -> Divide/1, To Workspace2/1
  Constant2/1 -> Divide/2
  Divide/1 -> To Workspace3/1
  Demux/1 -> MATLAB Function/5(phi)
  Demux/2 -> MATLAB Function/6(theta)
  Demux/3 -> Terminator/1
  Demux1/2 -> To Workspace4/1

== system Quad_Plant_dynamics/Quadcopter model/Force and Moment Calculation/Ground Model/Friction Force ==
  V : Inport
  Fn : Inport  Port=2
  Product : Product
  Saturation : Saturate  UpperLimit=contact.translation.maxFriction  LowerLimit=-contact.translation.maxFriction
  Soft Coulomb Friction : Subsystem
  Unary Minus : UnaryMinus
  Friction : Outport
  wires:
  Fn/1 -> Product/2
  Soft Coulomb Friction/1(Out1) -> Product/1
  Product/1 -> Unary Minus/1
  V/1 -> Soft Coulomb Friction/1(In1)
  Unary Minus/1 -> Saturation/1
  Saturation/1 -> Friction/1

== system Quad_Plant_dynamics/Quadcopter model/Force and Moment Calculation/Ground Model/Normal Force ==
  Vz : Inport
  Z : Inport  Port=2
  Add : Sum
  Constant : Constant  Value=0
  Damper Kp : Gain  Gain=-contact.translation.damper
  Saturation : Saturate  UpperLimit=contact.translation.maxNormal  LowerLimit=0
  Spring Kp : Gain  Gain=-contact.translation.spring
  Switch : Switch  Criteria=u2 > Threshold  SaturateOnIntegerOverflow=off  InputSameDT=off
  Unary Minus : UnaryMinus
  Unary Minus1 : UnaryMinus
  Normal : Outport
  wires:
  Constant/1 -> Switch/1
  Z/1 -> Unary Minus/1
  Switch/1 -> Saturation/1
  Damper Kp/1 -> Add/2
  Add/1 -> Switch/3
  Spring Kp/1 -> Add/1
  Vz/1 -> Unary Minus1/1
  Saturation/1 -> Normal/1
  Unary Minus/1 -> Spring Kp/1, Switch/2
  Unary Minus1/1 -> Damper Kp/1

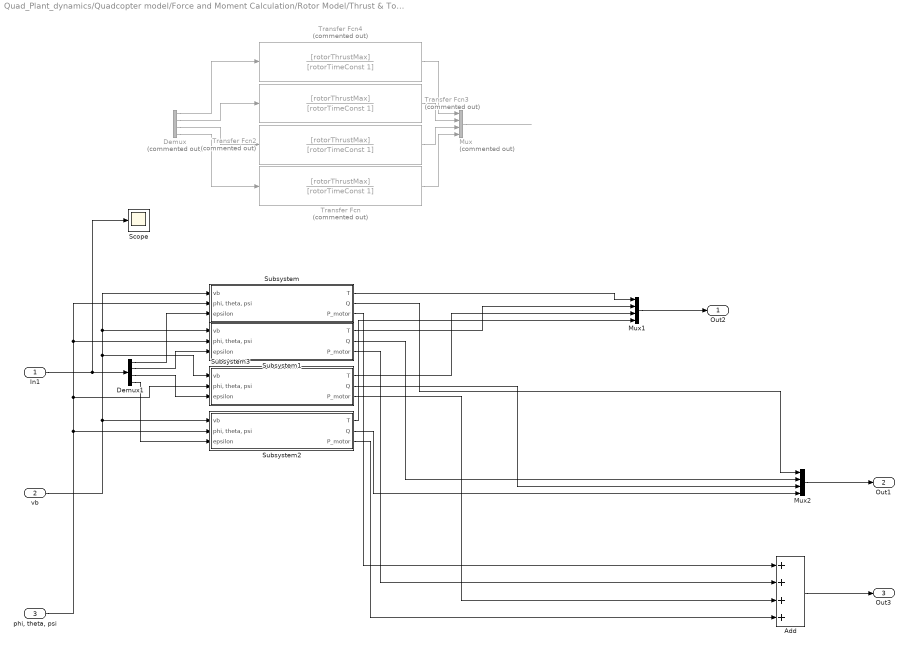
== system Quad_Plant_dynamics/Quadcopter model/Force and Moment Calculation/Rotor Model/Thrust & Torque model ==
  In1 : Inport
  vb : Inport  Port=2
  "phi, theta, psi" : Inport  Port=3
  Add : Sum  Inputs=++++
  Demux : Demux  Commented=on
  Demux1 : Demux
  Mux : Mux  Commented=on
  Mux1 : Mux
  Mux2 : Mux
  Scope : Scope
  Subsystem : Subsystem
  Subsystem1 : Subsystem
  Subsystem2 : Subsystem
  Subsystem3 : Subsystem
  Transfer Fcn{,2..4} (4 alike) : TransferFcn  Commented=on  Numerator=[rotorThrustMax]  Denominator=[rotorTimeConst 1]
  Out2 : Outport
  Out1 : Outport  Port=2
  Out3 : Outport  Port=3
  wires:
  Transfer Fcn3/1 -> Mux/2
  Demux/1 -> Transfer Fcn4/1
  Transfer Fcn2/1 -> Mux/3
  Demux/3 -> Transfer Fcn2/1
  Mux/1 -> ?
  Transfer Fcn4/1 -> Mux/1
  Demux/4 -> Transfer Fcn/1
  Demux/2 -> Transfer Fcn3/1
  Transfer Fcn/1 -> Mux/4
  Demux1/4 -> Subsystem2/3(epsilon)
  Demux1/3 -> Subsystem3/3(epsilon)
  Demux1/1 -> Subsystem/3(epsilon)
  Demux1/2 -> Subsystem1/3(epsilon)
  Subsystem/1(T) -> Mux1/1
  Subsystem2/1(T) -> Mux1/4
  Mux1/1 -> Out2/1
  Subsystem3/1(T) -> Mux1/3
  Subsystem1/1(T) -> Mux1/2
  Subsystem/2(Q) -> Mux2/1
  Subsystem2/2(Q) -> Mux2/4
  Mux2/1 -> Out1/1
  Subsystem3/2(Q) -> Mux2/3
  Subsystem1/2(Q) -> Mux2/2
  Subsystem/3(P_motor) -> Add/1
  Subsystem1/3(P_motor) -> Add/2
  Subsystem3/3(P_motor) -> Add/3
  Subsystem2/3(P_motor) -> Add/4
  Add/1 -> Out3/1
  vb/1 -> Subsystem3/1(vb), Subsystem/1(vb), Subsystem1/1(vb), Subsystem2/1(vb)
  "phi, theta, psi"/1 -> Subsystem3/2("phi, theta, psi"), Subsystem1/2("phi, theta, psi"), Subsystem/2("phi, theta, psi"), Subsystem2/2("phi, theta, psi")
  In1/1 -> Scope/1, Demux1/1

== system Quad_Plant_dynamics/Quadcopter model/Force and Moment Calculation/Rotor Model/Torque model ==
  In1 : Inport
  Demux : Demux
  Mux : Mux
  Transfer Fcn{1..4} (4 alike) : TransferFcn  Numerator=[rotorTorqueMax]  Denominator=[rotorTimeConst 1]
  Out1 : Outport
  wires:
  Transfer Fcn4/1 -> Mux/4
  Transfer Fcn3/1 -> Mux/3
  Transfer Fcn2/1 -> Mux/2
  Demux/2 -> Transfer Fcn2/1
  Demux/4 -> Transfer Fcn4/1
  Demux/3 -> Transfer Fcn3/1
  Mux/1 -> Out1/1
  Transfer Fcn1/1 -> Mux/1
  In1/1 -> Demux/1
  Demux/1 -> Transfer Fcn1/1

== system Quad_Plant_dynamics/Quadcopter model/Force and Moment Calculation/Ground Model/Friction Force/Soft Coulomb Friction ==
  note: Pennestrì, E., Rossi, V., Salvini, P. et al. Review and comparison of dry friction force models. Nonlinear Dyn 83, 1785–1801 (2016). https://doi.org/10.1007/s11071-015-2485-3
  In1 : Inport
  Tanh : Trigonometry  Operator=tanh
  friction coefficient : Gain  Gain=contact.translation.friction
  vd : Gain  Gain=1/contact.translation.vd
  Out1 : Outport
  wires:
  In1/1 -> vd/1
  vd/1 -> Tanh/1
  Tanh/1 -> friction coefficient/1
  friction coefficient/1 -> Out1/1

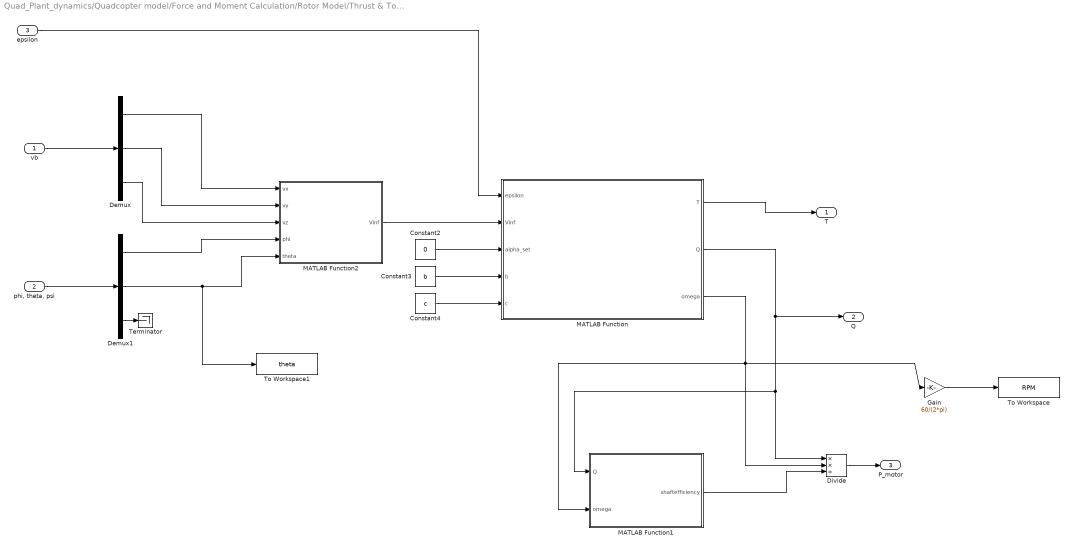
== system Quad_Plant_dynamics/Quadcopter model/Force and Moment Calculation/Rotor Model/Thrust & Torque model/Subsystem ==
  vb : Inport
  "phi, theta, psi" : Inport  Port=2
  epsilon : Inport  Port=3
  Constant2 : Constant  Value=0
  Constant3 : Constant  Value=b
  Constant4 : Constant  Value=c
  Demux : Demux  Outputs=3
  Demux1 : Demux  Outputs=3
  Divide : Product  Inputs=**/
  Gain : Gain  Gain=60/(2*pi)
  MATLAB Function : MATLAB Function  TreatAsAtomicUnit=on
  MATLAB Function1 : MATLAB Function  TreatAsAtomicUnit=on
  MATLAB Function2 : MATLAB Function  TreatAsAtomicUnit=on
  Terminator : Terminator
  To Workspace : ToWorkspace  VariableName=RPM  SaveFormat=Timeseries  SampleTime=-1
  To Workspace1 : ToWorkspace  VariableName=theta  SampleTime=-1
  T : Outport
  Q : Outport  Port=2
  P_motor : Outport  Port=3
  wires:
  MATLAB Function/2(Q) -> Q/1, MATLAB Function1/1(Q), Divide/1
  Demux/3 -> MATLAB Function2/3(vz)
  Constant2/1 -> MATLAB Function/3(alpha_set)
  Demux1/3 -> Terminator/1
  Demux/2 -> MATLAB Function2/2(vy)
  MATLAB Function/3(omega) -> Divide/2, Gain/1, MATLAB Function1/2(omega)
  vb/1 -> Demux/1
  Constant3/1 -> MATLAB Function/4(b)
  Demux1/1 -> MATLAB Function2/4(phi)
  MATLAB Function1/1(shaftefficiency) -> Divide/3
  Divide/1 -> P_motor/1
  Constant4/1 -> MATLAB Function/5(c)
  MATLAB Function/1(T) -> T/1
  "phi, theta, psi"/1 -> Demux1/1
  Demux1/2 -> To Workspace1/1, MATLAB Function2/5(theta)
  Demux/1 -> MATLAB Function2/1(vx)
  MATLAB Function2/1(Vinf) -> MATLAB Function/2(Vinf)
  epsilon/1 -> MATLAB Function/1(epsilon)
  Gain/1 -> To Workspace/1

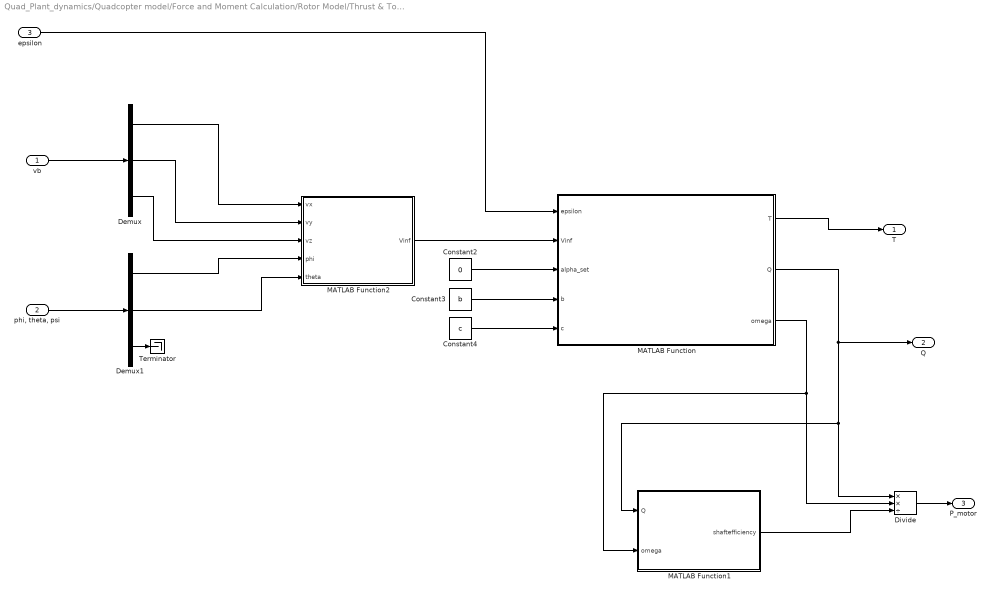
== system Quad_Plant_dynamics/Quadcopter model/Force and Moment Calculation/Rotor Model/Thrust & Torque model/Subsystem1 ==
  vb : Inport
  "phi, theta, psi" : Inport  Port=2
  epsilon : Inport  Port=3
  Constant2 : Constant  Value=0
  Constant3 : Constant  Value=b
  Constant4 : Constant  Value=c
  Demux : Demux  Outputs=3
  Demux1 : Demux  Outputs=3
  Divide : Product  Inputs=**/
  MATLAB Function : MATLAB Function  TreatAsAtomicUnit=on
  MATLAB Function1 : MATLAB Function  TreatAsAtomicUnit=on
  MATLAB Function2 : MATLAB Function  TreatAsAtomicUnit=on
  Terminator : Terminator
  T : Outport
  Q : Outport  Port=2
  P_motor : Outport  Port=3
  wires:
  MATLAB Function/2(Q) -> Q/1, MATLAB Function1/1(Q), Divide/1
  Demux/3 -> MATLAB Function2/3(vz)
  Constant2/1 -> MATLAB Function/3(alpha_set)
  Demux1/3 -> Terminator/1
  Demux/2 -> MATLAB Function2/2(vy)
  MATLAB Function/3(omega) -> Divide/2, MATLAB Function1/2(omega)
  epsilon/1 -> MATLAB Function/1(epsilon)
  vb/1 -> Demux/1
  Constant3/1 -> MATLAB Function/4(b)
  Demux1/1 -> MATLAB Function2/4(phi)
  MATLAB Function1/1(shaftefficiency) -> Divide/3
  Divide/1 -> P_motor/1
  Constant4/1 -> MATLAB Function/5(c)
  MATLAB Function2/1(Vinf) -> MATLAB Function/2(Vinf)
  MATLAB Function/1(T) -> T/1
  "phi, theta, psi"/1 -> Demux1/1
  Demux1/2 -> MATLAB Function2/5(theta)
  Demux/1 -> MATLAB Function2/1(vx)

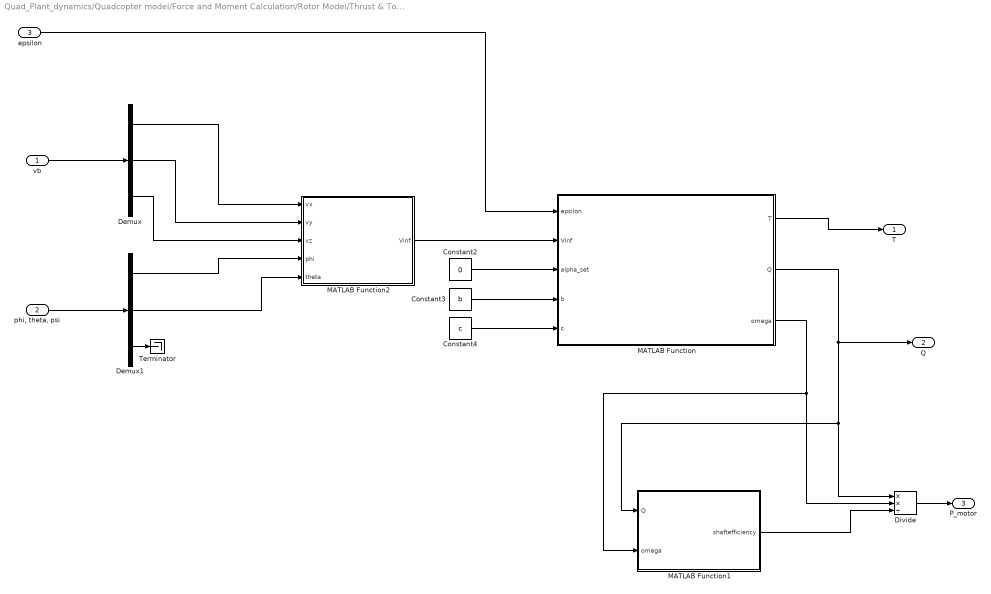
== system Quad_Plant_dynamics/Quadcopter model/Force and Moment Calculation/Rotor Model/Thrust & Torque model/Subsystem2 ==
  vb : Inport
  "phi, theta, psi" : Inport  Port=2
  epsilon : Inport  Port=3
  Constant2 : Constant  Value=0
  Constant3 : Constant  Value=b
  Constant4 : Constant  Value=c
  Demux : Demux  Outputs=3
  Demux1 : Demux  Outputs=3
  Divide : Product  Inputs=**/
  MATLAB Function : MATLAB Function  TreatAsAtomicUnit=on
  MATLAB Function1 : MATLAB Function  TreatAsAtomicUnit=on
  MATLAB Function2 : MATLAB Function  TreatAsAtomicUnit=on
  Terminator : Terminator
  T : Outport
  Q : Outport  Port=2
  P_motor : Outport  Port=3
  wires:
  MATLAB Function/2(Q) -> Q/1, MATLAB Function1/1(Q), Divide/1
  Demux/3 -> MATLAB Function2/3(vz)
  Constant2/1 -> MATLAB Function/3(alpha_set)
  Demux1/3 -> Terminator/1
  Demux/2 -> MATLAB Function2/2(vy)
  MATLAB Function/3(omega) -> Divide/2, MATLAB Function1/2(omega)
  epsilon/1 -> MATLAB Function/1(epsilon)
  vb/1 -> Demux/1
  Constant3/1 -> MATLAB Function/4(b)
  Demux1/1 -> MATLAB Function2/4(phi)
  MATLAB Function1/1(shaftefficiency) -> Divide/3
  Divide/1 -> P_motor/1
  Constant4/1 -> MATLAB Function/5(c)
  MATLAB Function2/1(Vinf) -> MATLAB Function/2(Vinf)
  MATLAB Function/1(T) -> T/1
  "phi, theta, psi"/1 -> Demux1/1
  Demux1/2 -> MATLAB Function2/5(theta)
  Demux/1 -> MATLAB Function2/1(vx)

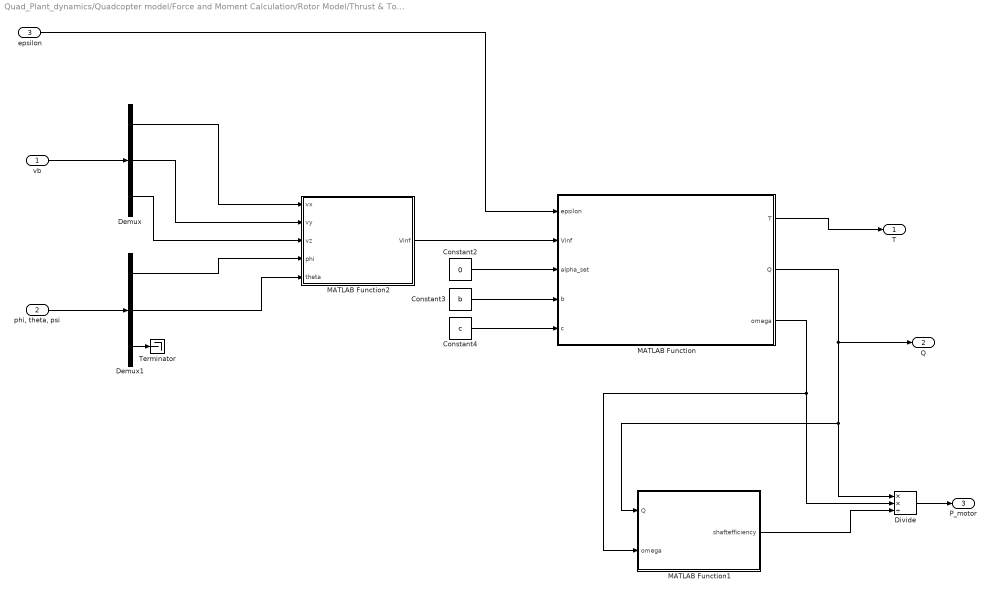
== system Quad_Plant_dynamics/Quadcopter model/Force and Moment Calculation/Rotor Model/Thrust & Torque model/Subsystem3 ==
  vb : Inport
  "phi, theta, psi" : Inport  Port=2
  epsilon : Inport  Port=3
  Constant2 : Constant  Value=0
  Constant3 : Constant  Value=b
  Constant4 : Constant  Value=c
  Demux : Demux  Outputs=3
  Demux1 : Demux  Outputs=3
  Divide : Product  Inputs=**/
  MATLAB Function : MATLAB Function  TreatAsAtomicUnit=on
  MATLAB Function1 : MATLAB Function  TreatAsAtomicUnit=on
  MATLAB Function2 : MATLAB Function  TreatAsAtomicUnit=on
  Terminator : Terminator
  T : Outport
  Q : Outport  Port=2
  P_motor : Outport  Port=3
  wires:
  MATLAB Function/2(Q) -> Q/1, MATLAB Function1/1(Q), Divide/1
  Demux/3 -> MATLAB Function2/3(vz)
  Constant2/1 -> MATLAB Function/3(alpha_set)
  Demux1/3 -> Terminator/1
  Demux/2 -> MATLAB Function2/2(vy)
  MATLAB Function/3(omega) -> Divide/2, MATLAB Function1/2(omega)
  epsilon/1 -> MATLAB Function/1(epsilon)
  vb/1 -> Demux/1
  Constant3/1 -> MATLAB Function/4(b)
  Demux1/1 -> MATLAB Function2/4(phi)
  MATLAB Function1/1(shaftefficiency) -> Divide/3
  Divide/1 -> P_motor/1
  Constant4/1 -> MATLAB Function/5(c)
  MATLAB Function2/1(Vinf) -> MATLAB Function/2(Vinf)
  MATLAB Function/1(T) -> T/1
  "phi, theta, psi"/1 -> Demux1/1
  Demux1/2 -> MATLAB Function2/5(theta)
  Demux/1 -> MATLAB Function2/1(vx)

== matlab function Quad_Plant_dynamics/Quadcopter model/Force and Moment Calculation/Rotor Model/Thrust & Torque model/Subsystem2/MATLAB Function ==
  settings: updateMethod=DISCRETE
  data: epsilon input; T output; Vinf input; alpha_set input; b input; c input; Q output; omega output
function [T, Q, omega]= BET(epsilon, Vinf, alpha_set, b, c)         
    
    omega=epsilon*837.758041+1e-6; 
    %air density
    rho=1.225;

    %angles
    theta=atan(0.1016./(2.*pi.*b));


    deltaT=zeros(10, length(b));
    deltaQ=deltaT;

%   while isreal(deltaT)==0
        for i=1:length(b)
  
            A= 0;%randi(3000)*0.0001; %initial guess for the axial inflow factor
            B= 0;%randi(3000)*0.0001; %initial guess for the swirl factor
            if i==1 || i==22
                dr=0.5*(b(2)-b(1));
            else
                dr=b(2)-b(1);
            end
            for j=1:10
                V0=Vinf*(1+A);
                V2=omega*b(i)*(1-B);
                V1=sqrt(V0^2+V2^2);
                alpha=atan(V0/V2);
                phi=theta(i)+alpha_set-alpha;
                % Cl=CL(phi);
                % Cd=CD(phi);
                phideg=rad2deg(phi);
                if phideg<=7.7
                    cl=0.1022*phideg+0.3749;
                elseif phideg>7.7 && phideg<=20
                    cl=0.0000118782*phideg^5-0.0006558208*phideg^4+0.0133404539* phideg^3-0.1264259735* phideg^2+0.6181804301*phideg-0.2152921158;
                else %phideg>20
                    cl=1.3805-1.3805*phideg/70;
                end
                alphadata=-8:1:19;
                CDdata=4.*[0.091 0.0838 0.0749 0.06 0.0305 0.028 0.0234 0.02 0.018 0.0174 0.0168 0.018 0.0186 0.0192 0.0197 0.022 0.0234 0.0251 0.0275 0.0317 0.0377 0.0455 0.0604 0.074 0.0868 0.108 0.1437 0.223];
                phideg=rad2deg(phi);
                if phideg>=-8 && phideg<=19
                    dragcoefficient=interp1(alphadata, CDdata, phideg);
                elseif phideg>19
                    dragcoefficient=0.892+(phideg-19)*0.016;
                else %phideg<-8
                    dragcoefficient=0.346+(-phideg-8)*0.02;
                end 
                Cl=cl;
                Cd=dragcoefficient;
                deltaT(j, i)=real(rho*V1^2*c(i)*(Cl*cos(alpha)-Cd*sin(alpha))*dr);
                deltaQ(j, i)=real(rho*V1^2*c(i)*(Cl*sin(alpha)+Cd*cos(alpha))*dr*b(i));
                % S=(pi*(b(i)+0.5*dr)^2)-(pi*(b(i)-0.5*dr)^2);
                % if Vinf~=0
                %     Btemp=deltaQ(j ,i)/(4*pi*b(i)^3*Vinf*(1+A)*omega*dr);
                %     Atemp=(-2*S*rho*Vinf^2+sqrt(4*S^2*rho^2*Vinf^4+8*deltaT(j, i)*S*rho*Vinf^2))/(4*S*rho*Vinf^2);
                % else
                %     Atemp=A;
                %     Btemp=B;
                % 
                % end    
                % A=0.5*(A+Atemp);
                % B=0.5*(B+Btemp);
            end
        end
%         if isreal(deltaT)==1
%             break
%         end
%     end

Ttemp=deltaT(10, :);
Qtemp=deltaQ(10, :);
T=real(sum(Ttemp));
Q=real(sum(Qtemp));
% M=sum(Mtemp);
% prop=T*Vinf/(omega*Q)
% zetashaft(Q, omega)
end

== matlab function Quad_Plant_dynamics/Quadcopter model/Force and Moment Calculation/Rotor Model/Thrust & Torque model/Subsystem2/MATLAB Function1 ==
  data: Q input; shaftefficiency output; omega input
function shaftefficiency=zetashaft(Q, omega)
    Kv=880;
    Kv=Kv*2*pi/60;
    Kt=1/Kv;
    R=0.108;
    Id=0.8; %drain current
    Vd=R*Id; %drain voltage
    VRPM=omega/Kv;
    I=Q/Kt;
    Vr=I*R;
    shaftefficiency=Q*omega/((VRPM+Vr+Vd)*(I+Id));
end

== matlab function Quad_Plant_dynamics/Quadcopter model/Force and Moment Calculation/Rotor Model/Thrust & Torque model/Subsystem2/MATLAB Function2 ==
  data: vx input; Vinf output; vy input; vz input; phi input; theta input
function Vinf = inflowspeed(vx, vy, vz, phi, theta)
    vxContribution=vx*sin(theta);
    vyContribution=vy*sin(phi);
    vzContribution=vz*cos(theta)*cos(phi);
    Vinf=sqrt(vxContribution^2+vyContribution^2+vzContribution^2);

== matlab function Quad_Plant_dynamics/Quadcopter model/Force and Moment Calculation/Rotor Model/Thrust & Torque model/Subsystem3/MATLAB Function ==
  settings: updateMethod=DISCRETE
  data: epsilon input; T output; Vinf input; alpha_set input; b input; c input; Q output; omega output
function [T, Q, omega]= BET(epsilon, Vinf, alpha_set, b, c)         
    
    omega=epsilon*837.758041+1e-6; 
    %air density
    rho=1.225;

    %angles
    theta=atan(0.1016./(2.*pi.*b));


    deltaT=zeros(10, length(b));
    deltaQ=deltaT;

%   while isreal(deltaT)==0
        for i=1:length(b)
  
            A= 0;%randi(3000)*0.0001; %initial guess for the axial inflow factor
            B= 0;%randi(3000)*0.0001; %initial guess for the swirl factor
            if i==1 || i==22
                dr=0.5*(b(2)-b(1));
            else
                dr=b(2)-b(1);
            end
            for j=1:10
                V0=Vinf*(1+A);
                V2=omega*b(i)*(1-B);
                V1=sqrt(V0^2+V2^2);
                alpha=atan(V0/V2);
                phi=theta(i)+alpha_set-alpha;
                % Cl=CL(phi);
                % Cd=CD(phi);
                phideg=rad2deg(phi);
                if phideg<=7.7
                    cl=0.1022*phideg+0.3749;
                elseif phideg>7.7 && phideg<=20
                    cl=0.0000118782*phideg^5-0.0006558208*phideg^4+0.0133404539* phideg^3-0.1264259735* phideg^2+0.6181804301*phideg-0.2152921158;
                else %phideg>20
                    cl=1.3805-1.3805*phideg/70;
                end
                alphadata=-8:1:19;
                CDdata=4.*[0.091 0.0838 0.0749 0.06 0.0305 0.028 0.0234 0.02 0.018 0.0174 0.0168 0.018 0.0186 0.0192 0.0197 0.022 0.0234 0.0251 0.0275 0.0317 0.0377 0.0455 0.0604 0.074 0.0868 0.108 0.1437 0.223];
                phideg=rad2deg(phi);
                if phideg>=-8 && phideg<=19
                    dragcoefficient=interp1(alphadata, CDdata, phideg);
                elseif phideg>19
                    dragcoefficient=0.892+(phideg-19)*0.016;
                else %phideg<-8
                    dragcoefficient=0.346+(-phideg-8)*0.02;
                end 
                Cl=cl;
                Cd=dragcoefficient;
                deltaT(j, i)=real(rho*V1^2*c(i)*(Cl*cos(alpha)-Cd*sin(alpha))*dr);
                deltaQ(j, i)=real(rho*V1^2*c(i)*(Cl*sin(alpha)+Cd*cos(alpha))*dr*b(i));
                % S=(pi*(b(i)+0.5*dr)^2)-(pi*(b(i)-0.5*dr)^2);
                % if Vinf~=0
                %     Btemp=deltaQ(j ,i)/(4*pi*b(i)^3*Vinf*(1+A)*omega*dr);
                %     Atemp=(-2*S*rho*Vinf^2+sqrt(4*S^2*rho^2*Vinf^4+8*deltaT(j, i)*S*rho*Vinf^2))/(4*S*rho*Vinf^2);
                % else
                %     Atemp=A;
                %     Btemp=B;
                % 
                % end    
                % A=0.5*(A+Atemp);
                % B=0.5*(B+Btemp);
            end
        end
%         if isreal(deltaT)==1
%             break
%         end
%     end

Ttemp=deltaT(10, :);
Qtemp=deltaQ(10, :);
T=real(sum(Ttemp));
Q=real(sum(Qtemp));
% M=sum(Mtemp);
% prop=T*Vinf/(omega*Q)
% zetashaft(Q, omega)
end

== matlab function Quad_Plant_dynamics/Quadcopter model/Force and Moment Calculation/Rotor Model/Thrust & Torque model/Subsystem3/MATLAB Function1 ==
  data: Q input; shaftefficiency output; omega input
function shaftefficiency=zetashaft(Q, omega)
    Kv=880;
    Kv=Kv*2*pi/60;
    Kt=1/Kv;
    R=0.108;
    Id=0.8; %drain current
    Vd=R*Id; %drain voltage
    VRPM=omega/Kv;
    I=Q/Kt;
    Vr=I*R;
    shaftefficiency=Q*omega/((VRPM+Vr+Vd)*(I+Id));
end

== matlab function Quad_Plant_dynamics/Quadcopter model/Force and Moment Calculation/Rotor Model/Thrust & Torque model/Subsystem/MATLAB Function1 ==
  data: Q input; shaftefficiency output; omega input
function shaftefficiency=zetashaft(Q, omega)
    Kv=880;
    Kv=Kv*2*pi/60;
    Kt=1/Kv;
    R=0.108;
    Id=0.8; %drain current
    Vd=R*Id; %drain voltage
    VRPM=omega/Kv;
    I=Q/Kt;
    Vr=I*R;
    shaftefficiency=Q*omega/((VRPM+Vr+Vd)*(I+Id));
end

== matlab function Quad_Plant_dynamics/Quadcopter model/Force and Moment Calculation/Rotor Model/Thrust & Torque model/Subsystem3/MATLAB Function2 ==
  data: vx input; Vinf output; vy input; vz input; phi input; theta input
function Vinf = inflowSpeed(vx, vy, vz, phi, theta)
    vxContribution=vx*sin(theta);
    vyContribution=vy*sin(phi);
    vzContribution=vz*cos(theta)*cos(phi);
    Vinf=sqrt(vxContribution^2+vyContribution^2+vzContribution^2);
